simulink model "Vehicle_Powertrain_Controller_1"  (R2014a)
settings: Solver=ode15s  StartTime=0.0  StopTime=100  RelTol=1e-3
PostLoadFcn:
  | num_fric_surf = 6;
  | eff_tor_rad = 0.4;
  | engagement_area = 0.0025;
  | peak_normal = 0.55;
  | fric_coeff = 0.5;
  | clutchRise = 0.1;
  | velTol = 1e-3;
  | pressThresh = 0.05;
  | p0 = 20e5;
libraries: sdl_lib x13, fl_lib x12, nesl_utility x9
Description:
  | Copyright 2014 The MathWorks, Inc.
settings Model: Creator=smiller  LastModifiedBy=smiller
settings DataIOCC: SignalLoggingSaveFormat=ModelDataLogs
settings OptimizationCC: ExpressionDepthLimit=2147483647
settings DebuggingCC: UnderspecifiedInitializationDetection=Classic  FcnCallInpInsideContextMsg=UseLocalSettings  StateNameClashWarn=warning
settings GRTTargetCC: CombineOutputUpdateFcns=off  GRTInterface=on

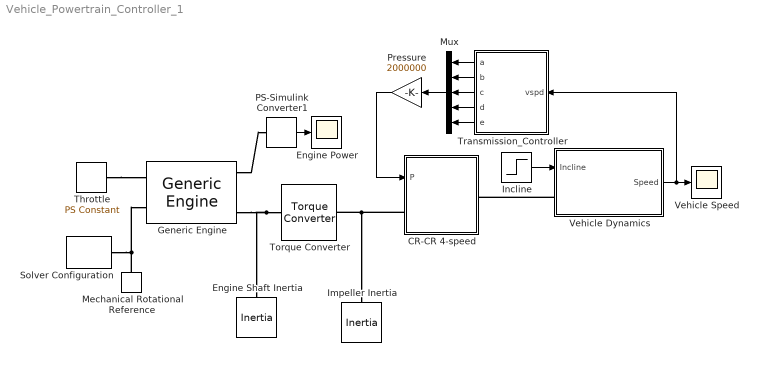
== system Vehicle_Powertrain_Controller_1 ==
  CR-CR 4-speed : Subsystem  mask(CR-CR 4-Speed){}
      mask help: This is a template for a CR-CR 4-speed transmission. Copy it to your model, open it as a subsystem, and modify it for your use.
      mask init:
      | drive_preinitmask(); Icon = drive_crcrgearblock('Mask');
      settings: OpenFcn=open_system(gcbh,'force');
      mask Help: web(drive_help);
      mask Display:
      | plot(Icon.x1,Icon.y1);
      | plot(Icon.x1_1,Icon.y1_1);
      | plot(Icon.x2,Icon.y2);
      | plot(Icon.x3,Icon.y3);
      | plot(Icon.x3_1,Icon.y3_1);
      | plot(Icon.x4,Icon.y4);
      | plot(Icon.x5,Icon.y5);
      | plot(Icon.x6,Icon.y6);
      | plot(Icon.x7,Icon.y7);
      | plot(Icon.x8,Icon.y8);
      | plot(Icon.x9,Icon.y9);
      | plot(Icon.x10,Icon.y10);
      | plot(Icon.x11,Icon.y11);
      | plot(Icon.x12,Icon.y12);
      | plot(Icon.x13,Icon.y13);
      | plot(Icon.x14,Icon.y14);
      | plot(Icon.x15,Icon.y15);
      | plot(Icon.x16,Icon.y16);
      | plot(Icon.x16_1,Icon.y16_1);
      | plot(Icon.x16_2,Icon.y16_2);
      | plot(Icon.x17,Icon.y17);
      | plot(Icon.x18,Icon.y18);
      | plot(Icon.x18_1,Icon.y18_1);
      | plot(Icon.x18_2,Icon.y18_2);
      | plot(Icon.x19,Icon.y19);
      | plot(Icon.x20,Icon.y20);
      | plot(Icon.x21,Icon.y21);
      | plot(Icon.x22,Icon.y22);
      | plot(Icon.x23,Icon.y23);
      | plot(Icon.x24,Icon.y24);
      | plot(Icon.x25,Icon.y25);
      | plot(Icon.x26,Icon.y26);
      | plot(Icon.x27,Icon.y27);
      | plot(Icon.x28,Icon.y28);
      | plot(Icon.x29,Icon.y29);
      | 
      | plot(Icon.LowerLeftx,Icon.LowerLefty);
      | plot(Icon.UpperRightx,Icon.UpperRighty);
  Engine Power : Scope
      settings: YMin=0  YMax=150000  SaveName=Simple_PT_Engine_DATA
  Engine Shaft Inertia : fl_lib/Mechanical/Rotational Elements/Inertia  inertia=0.2 kg*m^2  w_specify=on  w_priority=High  w=800 rpm  t_specify=off  t_priority=High  t=0 N*m
  Generic Engine : sdl_lib/Engines/Generic Engine  model_parameterization=1  engine_type=1  P_max=1.5e+5 W  w_P_max=4.5e+3 rpm  w_max=6e+3 rpm  w_min=500 rpm  w_tab=[ 500 1000 2e+3 3e+3 4e+3 5e+3 6e+3 7e+3 ] rpm  trq_tab=[ 380 380 380 380 350 280 200 80 ] N*m  pwr_tab=[ 2e+4 4e+4 7.8e+4 1.2e+5 1.45e+5 1.48e+5 1.25e+5 6e+4 ] W  interp_method=1  model_inertia=0  inertia=1 kg*m^2  initial_velocity=800 rpm  model_time_constant=0  time_constant=0.2 s  T0=0  w_thr=100 rpm  idle_speed=0  idle_speed_reference=1000 rpm  tau_controller=1 s  idle_w_thr=1 rpm  fc_model=1  fc_per_rev=25 mg/rev  displaced_volume=400 cm^3  rev_per_cycle=2  fc_w_tab=[ 1000 2e+3 3e+3 4e+3 5e+3 6e+3 ] rpm  fc_trq_tab=[ 0 80 160 200 240 320 360 400 ] N*m  fc_tab=[ 0.5 0.9 1.4 1.6 1.9 2.7 3.4 4.4; 1 1.7 2.7 3.1 3.6 5 6 7.4; 1.4 2.7 4 4.8 5.6 7.5 8.5 10.5; 2 3.6 5.8 6.7 8 10.4 11.7 13.3; 2.5 4.8 7.9 9.4 10.8 14 16.2 18.6; 3.1 6 10.3 11.9 13.8 18.4 22 26.5 ] g/s  bmep_tab=[ 0 250 500 625 750 1000 1.15e+3 1.25e+3 ] kPa  bsfc_tab=[ 410 380 300 280 270 290 320 380; 410 370 290 270 260 270 285 320; 415 380 290 275 265 270 270 300; 420 390 310 290 285 280 280 285; 430 410 340 320 310 300 310 320; 450 430 370 340 330 330 350 380 ] g/hr/kW  fc_interp_method=1
  Impeller Inertia : fl_lib/Mechanical/Rotational Elements/Inertia  inertia=1 kg*m^2  w_specify=on  w_priority=High  w=0 rpm  t_specify=off  t_priority=High  t=0 N*m
  Incline : Step  Time=5  After=20  SampleTime=0
  Mechanical Rotational Reference : fl_lib/Mechanical/Rotational Elements/Mechanical Rotational Reference
  Mux : Mux  Inputs=5
  PS-Simulink Converter1 : nesl_utility/PS-Simulink Converter  PhysicalDomain=network_engine_domain  SubClassName=ps_output  LeftPortType=input  RightPortType=output  PseudoPeriodic=off  Frequencies=[]  Unit=W  AffineConversion=off
  Pressure : Gain  Gain=2000000
  Solver Configuration : nesl_utility/Solver Configuration  PhysicalDomain=network_engine_domain  SubClassName=solver  LeftPortType=input  RightPortType=generic  Accelerate=off  Tones=[]  Harmonics=[]  SimulateNoise=off  Profile=off  UseLocalSampling=off  EnableSwitchedLinearOptims=on  FrequencyDomain=off  UseCCode=off  RelTol=0.001  AbsTol=1e-06  MinStep=1e-09  ToWorkspace=off  DoDC=off  ResidualTolerance=1e-9  UseLocalSolver=off  LocalSolverChoice=NE_BACKWARD_EULER_ADVANCER  LocalSolverSampleTime=.001  DoFixedCost=off  MaxNonlinIter=3  MaxModeIter=2  LinearAlgebra=Sparse  DelaysMemoryBudget=1024  AutomaticFiltering=on  FilteringTimeConstant=0.001
  Throttle : fl_lib/Physical Signals/Sources/PS Constant  constant=0.5
  Torque Converter : sdl_lib/Couplings & Drives/Torque Converter  n_vector=[ 0 0.5 0.6 0.7 0.8 0.81 0.82 0.83 0.84 0.85 0.86 0.87 0.88 0.89 0.9 0.92 0.94 0.96 0.97 ]  trq_vector=[ 2.232 1.5462 1.4058 1.2746 1.1528 1.1412 1.1296 1.1181 1.1067 1.0955 1.0843 1.0732 1.0622 1.0513 1.0405 1.0192 0.9983 0.9983 0.9983 ]  cf_vector_parameterization=1  cf_vector_reference_speed=1  cf_vector=[ 12.2938 12.8588 13.1452 13.6285 14.6163 14.7747 14.9516 15.1502 15.3748 15.6309 15.9253 16.2675 16.6698 17.1492 17.7298 19.3503 22.1046 29.9986 50 ] (rad/s)/(N*m)^0.5  cf_vector_sq=[ 0.006615999999999999 0.006048 0.005787 0.005384 0.004681 0.004581 0.004473 0.004357 0.00423 0.004093 0.003943 0.003779 0.003599 0.0034 0.003181 0.002671 0.002047 0.001111 4e-4 ] N*m/(rad/s)^2  interp_method=1  extrap_method=1  model_lag=0  tau=0.02 s  initial_trq_ratio=0
  Transmission_Controller : Stateflow chart  TreatAsAtomicUnit=on
  Vehicle Dynamics : Subsystem
  Vehicle Speed : Scope
      settings: YMin=-10  YMax=90  SaveName=Simple_PT_Speed_DATA
  wires:
  Vehicle Dynamics/1(Speed) -> Vehicle Speed/1, Transmission_Controller/1(vspd)
  PS-Simulink Converter1/1 -> Engine Power/1
  Incline/1 -> Vehicle Dynamics/1(Incline)
  Transmission_Controller/2(b) -> Mux/2
  Transmission_Controller/3(c) -> Mux/3
  Transmission_Controller/4(d) -> Mux/4
  Transmission_Controller/5(e) -> Mux/5
  Mux/1 -> Pressure/1
  Pressure/1 -> CR-CR 4-speed/1(P)
  Transmission_Controller/1(a) -> Mux/1
  connections:
  Mechanical Rotational Reference/LConn1 -- Generic Engine/LConn2 -- Solver Configuration/RConn1
  Vehicle Dynamics/LConn1 -- CR-CR 4-speed/RConn1
  Throttle/RConn1 -- Generic Engine/LConn1
  CR-CR 4-speed/LConn1 -- Torque Converter/RConn1 -- Impeller Inertia/LConn1
  Generic Engine/RConn1 -- PS-Simulink Converter1/LConn1
  Torque Converter/LConn1 -- Engine Shaft Inertia/LConn1 -- Generic Engine/RConn3

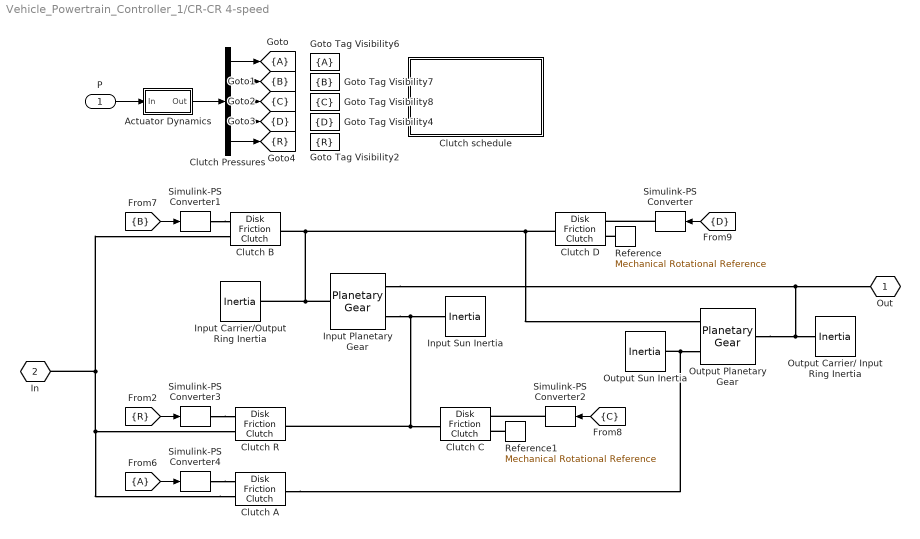
== system Vehicle_Powertrain_Controller_1/CR-CR 4-speed ==
  P : Inport
  Actuator Dynamics : Subsystem  mask(First-order lag supporting vector signals){b=clutchRise, x_initial=0}
      mask prompts: b "Filter time constant"; x_initial "Initial output"
      mask help: Models a lag of the form 1/(b*s+1) where s is the Laplace operator.
  Clutch Pressures : Demux  Outputs=5
  Clutch schedule : Subsystem
      mask Display: fprintf('Double-click to show\n Clutch Schedule')
  Clutch A : sdl_lib/Clutches/Disk Friction Clutch  geometry_model=1  r_eff=eff_tor_rad m  d_o=0.15 m  d_i=0.1 m  nS=num_fric_surf  piston_area=engagement_area m^2  friction_model=1  mu_coulomb=fric_coeff  mu_w_vector=[ 0 0.1 0.2 0.3 0.4 0.5 1 2 5 10 100 1000 ] rad/s  mu_coulomb_vector=[ 0.29 0.28 0.26 0.22 0.21 0.2 0.2 0.19 0.19 0.19 0.19 0.19 ]  mu_interp_method=1  mu_extrap_method=1  mu_static=peak_normal  d_f=1  w_tol=velTol rad/s  pressure_min=pressThresh*p0 Pa  mu_visc=0 N*m/(rad/s)  initial_state_locked=1
  Clutch B : sdl_lib/Clutches/Disk Friction Clutch  geometry_model=1  r_eff=eff_tor_rad m  d_o=0.15 m  d_i=0.1 m  nS=num_fric_surf  piston_area=engagement_area m^2  friction_model=1  mu_coulomb=fric_coeff  mu_w_vector=[ 0 0.1 0.2 0.3 0.4 0.5 1 2 5 10 100 1000 ] rad/s  mu_coulomb_vector=[ 0.29 0.28 0.26 0.22 0.21 0.2 0.2 0.19 0.19 0.19 0.19 0.19 ]  mu_interp_method=1  mu_extrap_method=1  mu_static=peak_normal  d_f=1  w_tol=velTol rad/s  pressure_min=pressThresh*p0 Pa  mu_visc=0 N*m/(rad/s)  initial_state_locked=0
  Clutch C : sdl_lib/Clutches/Disk Friction Clutch  geometry_model=1  r_eff=eff_tor_rad m  d_o=0.15 m  d_i=0.1 m  nS=num_fric_surf  piston_area=engagement_area m^2  friction_model=1  mu_coulomb=fric_coeff  mu_w_vector=[ 0 0.1 0.2 0.3 0.4 0.5 1 2 5 10 100 1000 ] rad/s  mu_coulomb_vector=[ 0.29 0.28 0.26 0.22 0.21 0.2 0.2 0.19 0.19 0.19 0.19 0.19 ]  mu_interp_method=1  mu_extrap_method=1  mu_static=peak_normal  d_f=1  w_tol=velTol rad/s  pressure_min=pressThresh*p0 Pa  mu_visc=0 N*m/(rad/s)  initial_state_locked=0
  Clutch D : sdl_lib/Clutches/Disk Friction Clutch  geometry_model=1  r_eff=eff_tor_rad m  d_o=0.15 m  d_i=0.1 m  nS=num_fric_surf  piston_area=engagement_area m^2  friction_model=1  mu_coulomb=fric_coeff  mu_w_vector=[ 0 0.1 0.2 0.3 0.4 0.5 1 2 5 10 100 1000 ] rad/s  mu_coulomb_vector=[ 0.29 0.28 0.26 0.22 0.21 0.2 0.2 0.19 0.19 0.19 0.19 0.19 ]  mu_interp_method=1  mu_extrap_method=1  mu_static=peak_normal  d_f=1  w_tol=velTol rad/s  pressure_min=pressThresh*p0 Pa  mu_visc=0 N*m/(rad/s)  initial_state_locked=1
  Clutch R : sdl_lib/Clutches/Disk Friction Clutch  geometry_model=1  r_eff=eff_tor_rad m  d_o=0.15 m  d_i=0.1 m  nS=num_fric_surf  piston_area=engagement_area m^2  friction_model=1  mu_coulomb=fric_coeff  mu_w_vector=[ 0 0.1 0.2 0.3 0.4 0.5 1 2 5 10 100 1000 ] rad/s  mu_coulomb_vector=[ 0.29 0.28 0.26 0.22 0.21 0.2 0.2 0.19 0.19 0.19 0.19 0.19 ]  mu_interp_method=1  mu_extrap_method=1  mu_static=peak_normal  d_f=1  w_tol=velTol rad/s  pressure_min=pressThresh*p0 Pa  mu_visc=0 N*m/(rad/s)  initial_state_locked=0
  Goto Tag Visibility2 : GotoTagVisibility  GotoTag=R
  Goto Tag Visibility4 : GotoTagVisibility  GotoTag=D
  Goto Tag Visibility6 : GotoTagVisibility
  Goto Tag Visibility7 : GotoTagVisibility  GotoTag=B
  Goto Tag Visibility8 : GotoTagVisibility  GotoTag=C
  "Input Planetary Gear " : sdl_lib/Gears/Planetary Gear  rs_ratio=2.2258  friction_model=1  efficiency=[ 0.96 0.98 ]  mu_visc=[ 0 0 ] N*m/(rad/s)  w_thr=[ 0.01 0.01 ] rad/s
  Input Carrier/Output Ring Inertia : fl_lib/Mechanical/Rotational Elements/Inertia  inertia=1e-4 kg*m^2  w_specify=on  w_priority=High  w=0 rad/s  t_specify=off  t_priority=High  t=0 N*m
  Input Sun Inertia : fl_lib/Mechanical/Rotational Elements/Inertia  inertia=1e-4 kg*m^2  w_specify=on  w_priority=High  w=0 rad/s  t_specify=off  t_priority=High  t=0 N*m
  Output Planetary Gear : sdl_lib/Gears/Planetary Gear  rs_ratio=1.84  friction_model=1  efficiency=[ 0.96 0.98 ]  mu_visc=[0 0] N*m/(rad/s)  w_thr=[ 0.01 0.01 ] rad/s
  "Output Carrier/ Input Ring Inertia " : fl_lib/Mechanical/Rotational Elements/Inertia  inertia=1e-4 kg*m^2  w_specify=on  w_priority=High  w=0 rad/s  t_specify=off  t_priority=High  t=0 N*m
  Output Sun Inertia : fl_lib/Mechanical/Rotational Elements/Inertia  inertia=1e-4 kg*m^2  w_specify=on  w_priority=High  w=0 rad/s  t_specify=off  t_priority=High  t=0 N*m
  Reference : fl_lib/Mechanical/Rotational Elements/Mechanical Rotational Reference
  Reference1 : fl_lib/Mechanical/Rotational Elements/Mechanical Rotational Reference
  Simulink-PS Converter{,1..4} (5 alike) : nesl_utility/Simulink-PS Converter  PhysicalDomain=network_engine_domain  SubClassName=ps_input  LeftPortType=input  RightPortType=output  PseudoPeriodic=off  Frequencies=[]  NoiseDistribution=none  NoiseParameters=[]  Unit=1  AffineConversion=off  InputFiltering=off  SimscapeFilterOrder=1  InputFilterTimeConstant=.001  UdotUserProvided=0
  Out : PMIOPort  Tag=PMCPort  Port=1  Side=Right
  In : PMIOPort  Tag=PMCPort  Port=2  Side=Left
  tag scope: A=scoped, B=scoped, C=scoped, D=scoped, R=scoped
  wires:
  Actuator Dynamics/1(Out) -> Clutch Pressures/1
  P/1 -> Actuator Dynamics/1(In)
  Clutch Pressures/1 -> [A]
  Clutch Pressures/2 -> [B]
  Clutch Pressures/3 -> [C]
  Clutch Pressures/4 -> [D]
  Clutch Pressures/5 -> [R]
  [D] -> Simulink-PS Converter/1
  [B] -> Simulink-PS Converter1/1
  [C] -> Simulink-PS Converter2/1
  [R] -> Simulink-PS Converter3/1
  [A] -> Simulink-PS Converter4/1
  connections:
  "Input Planetary Gear "/RConn1 -- Output Planetary Gear/LConn1 -- "Output Carrier/ Input Ring Inertia "/LConn1 -- Out/RConn1
  Clutch A/RConn1 -- Output Planetary Gear/RConn2 -- Output Sun Inertia/LConn1
  Reference/LConn1 -- Clutch D/LConn2
  Simulink-PS Converter/RConn1 -- Clutch D/LConn1
  Clutch R/RConn1 -- "Input Planetary Gear "/RConn2 -- Input Sun Inertia/LConn1 -- Clutch C/RConn1
  Clutch B/RConn1 -- Output Planetary Gear/RConn1 -- Clutch D/RConn1 -- "Input Planetary Gear "/LConn1 -- Input Carrier/Output Ring Inertia/LConn1
  Simulink-PS Converter1/RConn1 -- Clutch B/LConn1
  Clutch A/LConn2 -- In/RConn1 -- Clutch B/LConn2 -- Clutch R/LConn2
  Reference1/LConn1 -- Clutch C/LConn2
  Simulink-PS Converter2/RConn1 -- Clutch C/LConn1
  Simulink-PS Converter3/RConn1 -- Clutch R/LConn1
  Simulink-PS Converter4/RConn1 -- Clutch A/LConn1

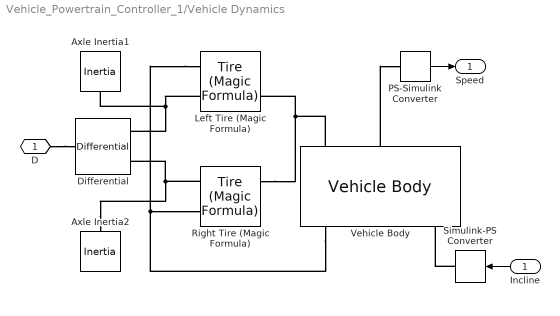
== system Vehicle_Powertrain_Controller_1/Vehicle Dynamics ==
  Incline : Inport
  Axle Inertia1 : fl_lib/Mechanical/Rotational Elements/Inertia  inertia=1 kg*m^2  w_specify=on  w_priority=High  w=0 rad/s  t_specify=off  t_priority=High  t=0 N*m
  Axle Inertia2 : fl_lib/Mechanical/Rotational Elements/Inertia  inertia=1 kg*m^2  w_specify=on  w_priority=High  w=0 rad/s  t_specify=off  t_priority=High  t=0 N*m
  Differential : sdl_lib/Gears/Differential  driveshaft_location=2  cd_ratio=4  friction_model=1  efficiency=[ 0.85 0.92 ]  mu_visc=[ 0 0 ] N*m/(rad/s)  w_thr=[ 0.01 0.01 ] rad/s
  Left Tire (Magic Formula) : sdl_lib/Tires & Vehicles/Tire (Magic Formula)  parameterization=1  F_z1=3e+3 N  F_x1=3.5e+3 N  kappa1=10  B_m=10  C_m=1.9  D_m=1  E_m=0.97  fz0=4e+3 N  p_Cx=1.685  p_Dx=[ 1.21 -0.037 ]  p_Ex=[ 0.344 0.095 -0.02 0 ]  p_Kx=[ 21.51 -0.163 0.245 ]  p_Hx=[ -0.002 0.002 ]  p_Vx=[ 0 0 ]  v_tr_thr=0.1 m/s  r_e=0.3 m  model_compliance=0  stiffness=1e+6 N/m  damping=1000 N/(m/s)  model_inertia=0  inertia=1 kg*m^2  initial_velocity=0 rad/s  model_resistance=0  resistance_model=1  coeff=0.015  p_tire=250e3 Pa  alpha=-0.003  beta=0.97  coeff_a=84e-4  coeff_b=6.2e-4 s/m  coeff_c=1.6e-4 s^2/m^2  v_thr=1e-3 m/s
  PS-Simulink Converter : nesl_utility/PS-Simulink Converter  PhysicalDomain=network_engine_domain  SubClassName=ps_output  LeftPortType=input  RightPortType=output  PseudoPeriodic=off  Frequencies=[]  Unit=km/hr  AffineConversion=off
  Right Tire (Magic Formula) : sdl_lib/Tires & Vehicles/Tire (Magic Formula)  parameterization=1  F_z1=3e+3 N  F_x1=3.5e+3 N  kappa1=10  B_m=10  C_m=1.9  D_m=1  E_m=0.97  fz0=4e+3 N  p_Cx=1.685  p_Dx=[ 1.21 -0.037 ]  p_Ex=[ 0.344 0.095 -0.02 0 ]  p_Kx=[ 21.51 -0.163 0.245 ]  p_Hx=[ -0.002 0.002 ]  p_Vx=[ 0 0 ]  v_tr_thr=0.1 m/s  r_e=0.3 m  model_compliance=0  stiffness=1e+6 N/m  damping=1000 N/(m/s)  model_inertia=0  inertia=1 kg*m^2  initial_velocity=0 rad/s  model_resistance=0  resistance_model=1  coeff=0.015  p_tire=250e3 Pa  alpha=-0.003  beta=0.97  coeff_a=84e-4  coeff_b=6.2e-4 s/m  coeff_c=1.6e-4 s^2/m^2  v_thr=1e-3 m/s
  Simulink-PS Converter : nesl_utility/Simulink-PS Converter  PhysicalDomain=network_engine_domain  SubClassName=ps_input  LeftPortType=input  RightPortType=output  PseudoPeriodic=off  Frequencies=[]  NoiseDistribution=none  NoiseParameters=[]  Unit=deg  AffineConversion=off  InputFiltering=off  SimscapeFilterOrder=1  InputFilterTimeConstant=.001  UdotUserProvided=0
  Vehicle Body : sdl_lib/Tires & Vehicles/Vehicle Body  mass=1.2e+3 kg  n_w=2  x_f=1.4 m  x_r=1.6 m  y_c=0.5 m  area=3 m^2  Cd=0.4  v0=0 m/s  g=9.81 m/s^2  rho=1.18 kg/m^3
  D : PMIOPort  Port=1  Side=Left
  Speed : Outport
  wires:
  PS-Simulink Converter/1 -> Speed/1
  Incline/1 -> Simulink-PS Converter/1
  connections:
  Axle Inertia1/LConn1 -- Left Tire (Magic Formula)/LConn2 -- Differential/RConn2
  Axle Inertia2/LConn1 -- Right Tire (Magic Formula)/LConn2 -- Differential/RConn1
  Left Tire (Magic Formula)/LConn1 -- Vehicle Body/RConn1 -- Right Tire (Magic Formula)/LConn1
  Vehicle Body/LConn1 -- Right Tire (Magic Formula)/RConn2 -- Left Tire (Magic Formula)/RConn2
  Vehicle Body/LConn2 -- PS-Simulink Converter/LConn1
  Simulink-PS Converter/RConn1 -- Vehicle Body/RConn3
  D/RConn1 -- Differential/LConn1

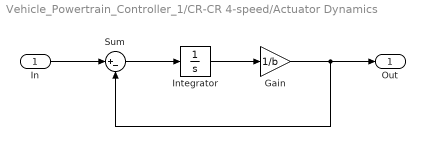
== system Vehicle_Powertrain_Controller_1/CR-CR 4-speed/Actuator Dynamics ==
  In : Inport
  Gain : Gain  Gain=1/b
  Integrator : Integrator  InitialCondition=x_initial
  Sum : Sum  Inputs=|+-  SaturateOnIntegerOverflow=on  InputSameDT=on  OutDataTypeStr=Inherit: Same as first input
  Out : Outport
  wires:
  Gain/1 -> Out/1, Sum/2
  Integrator/1 -> Gain/1
  In/1 -> Sum/1
  Sum/1 -> Integrator/1

== system Vehicle_Powertrain_Controller_1/CR-CR 4-speed/Clutch schedule ==
  note: F = Free
      | L = Locked
  note: g1: Ravigneaux ring (R)/large sun (S1) gear ratio
      | g2: Ravigneaux ring (R)/small sun (S2) gear ratio
  note: F
  note: F
  note: F
  note: F
  note: F
  note: L
  note: E
  note: D
  note: C
  note: B
  note: A
  note: Gear
  note: Clutch Schedule
  note: R
      |
      | 1
      |
      | 2
      |
      | 3
      |
      | 4
  note: F
  note: F
  note: F
  note: L
  note: Ratio
  note: L
  note: F
  note: L
  note: F
  note: F
  note: F
  note: L
  note: L
  note: L
  note: F
  note: L
  note: L
  note: F
  note: L
  note: F
  note: -g1
  note: g2
  note: (g1+g2)/(1+g1)
  note: 1
  note: g1/(1+g1)
  note: ---------------------------------------------------------------------------------------------------------------------------------------------------------------
  note: |
      | |
      | |
      | |
      | |
      | |
      | |
      | |
      | |
      | |
      | |
      | |
      | |
      | |
  note: |
      | |
      | |
      | |
      | |
      | |
      | |
      | |
      | |
      | |
      | |
      | |
      | |
      | |
  note: |
      | |
      | |
      | |
      | |
      | |
      | |
      | |
      | |
      | |
      | |
      | |
      | |
      | |
  note: |
      | |
      | |
      | |
      | |
      | |
      | |
      | |
      | |
      | |
      | |
      | |
      | |
      | |
  note: |
      | |
      | |
      | |
      | |
      | |
      | |
      | |
      | |
      | |
      | |
      | |
      | |
      | |
  note: |
      | |
      | |
      | |
      | |
      | |
      | |
      | |
      | |
      | |
      | |
      | |
      | |
      | |
  note: |
      | |
      | |
      | |
      | |
      | |
      | |
      | |
      | |
      | |
      | |
      | |
      | |
      | |
  note: ---------------------------------------------------------------------------------------------------------------------------------------------------------------
  note: ---------------------------------------------------------------------------------------------------------------------------------------------------------------
  note: |
      | |
      | |
      | |
      | |
      | |
      | |
      | |
      | |
      | |
      | |
      | |
      | |
      | |
  note: ---------------------------------------------------------------------------------------------------------------------------------------------------------------
  note: ---------------------------------------------------------------------------------------------------------------------------------------------------------------
  note: ---------------------------------------------------------------------------------------------------------------------------------------------------------------
  note: ---------------------------------------------------------------------------------------------------------------------------------------------------------------

== stateflow chart Vehicle_Powertrain_Controller_1/Transmission_Controller ==
  state first
    a=0;
    b=0;
    c=0;
    d=0;
    e=0;
  state third
    a=0;
    b=0;
    c=0;
    d=0;
    e=0;
  state second
    a=0;
    b=0;
    c=0;
    d=0;
    e=0;
  state fourth
    a=0;
    b=0;
    c=0;
    d=0;
    e=0;
  third -> fourth [order 1] : [vspd>100]
  first -> second : [vspd>30]
  second -> third [order 1] : [vspd>65]
  (default) -> first
  second -> first [order 2] : [vspd<20]
  third -> second [order 2] : [vspd<55]
  fourth -> third : [vspd<90]
  data: vspd input; a output double; b output double; c output double; d output double; e output double
